simulink model "Part1_170747"  (R2019a)
settings: Solver=ode2  StartTime=0.0  StopTime=700  FixedStep=0.1  RelTol=1e-3
undefined symbols (not defined in the file): D, Km, T
settings Model: Creator=HP  LastModifiedBy=singh
settings DataIOCC: ReturnWorkspaceOutputs=off
settings DebuggingCC: ArithmeticOperatorsInVariantConditions=warning

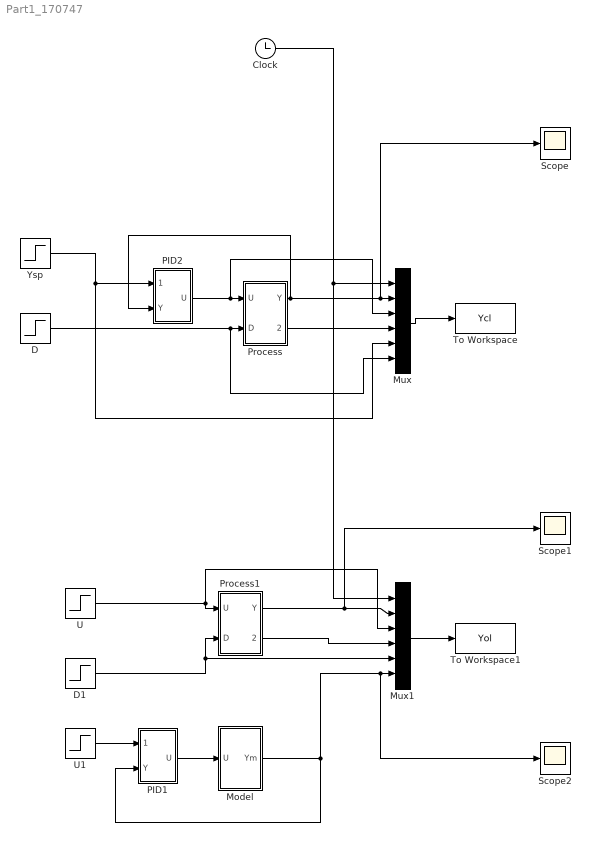
== system Part1_170747 ==
  Clock : Clock
  D : Step  Time=0  After=0  SampleTime=0
  D1 : Step  Time=0  After=0  SampleTime=0
  Model : Subsystem
  Mux : Mux  Inputs=6
  Mux1 : Mux  Inputs=6
  PID1 : Subsystem  mask{Kc=2.81, Ti=1e10, Td=0}
      mask prompts: Kc "Proportional Gain"; Ti "Integral Time"; Td "Derivative Time"
  PID2 : Subsystem  mask{Kc=3.4071/1.7, Ti=106.2/2, Td=106.2/8}
      mask prompts: Kc "Proportional Gain"; Ti "Integral Time"; Td "Derivative Time"
  Process : Subsystem  mask{K1=0.45, K2=0.45, T1=0.5, T2=0.5, K=1/17e-4}
      mask prompts: K1 "Forward Gain"; K2 "Rev Gain"; T1 "Forward Time Constt"; T2 "Rev Time Constt"; K "Scaling Gain"
  Process1 : Subsystem  mask{K1=0.45, K2=0.45, T1=0.5, T2=0.5, K=1/17e-4}
      mask prompts: K1 "Forward Gain"; K2 "Rev Gain"; T1 "Forward Time Constt"; T2 "Rev Time Constt"; K "Scaling Gain"
  Scope : Scope
  Scope1 : Scope
  Scope2 : Scope
  To Workspace : ToWorkspace  VariableName=Ycl  SampleTime=-1
  To Workspace1 : ToWorkspace  VariableName=Yol  SampleTime=-1
  U : Step  Time=0  SampleTime=0
  U1 : Step  Time=0  SampleTime=0
  Ysp : Step  Time=0  SampleTime=0
  wires:
  Clock/1 -> Mux/1, Mux1/1
  Process/1(Y) -> PID2/2(Y), Scope/1, Mux/2
  Process/2(Uimp) -> Mux/4
  Mux/1 -> To Workspace/1
  D/1 -> Mux/6, Process/2(D)
  Ysp/1 -> PID2/1(Ysp), Mux/5
  Mux1/1 -> To Workspace1/1
  U/1 -> Mux1/3, Process1/1(U)
  D1/1 -> Process1/2(D), Mux1/5
  Process1/1(Y) -> Mux1/2, Scope1/1
  PID2/1(U) -> Mux/3, Process/1(U)
  Process1/2(Uimp) -> Mux1/4
  Model/1("Ym ") -> Scope2/1, Mux1/6, PID1/2(Y)
  PID1/1(U) -> Model/1(U)
  U1/1 -> PID1/1(Ysp)

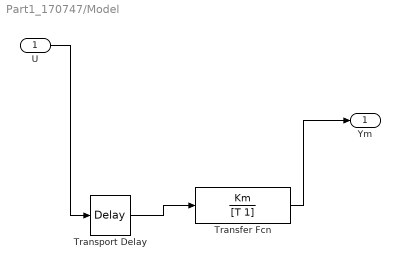
== system Part1_170747/Model ==
  U : Inport
  Transfer Fcn : TransferFcn  Numerator=Km  Denominator=[T 1]
  Transport Delay : TransportDelay  DelayTime=D
  "Ym " : Outport
  wires:
  Transport Delay/1 -> Transfer Fcn/1
  Transfer Fcn/1 -> "Ym "/1
  U/1 -> Transport Delay/1

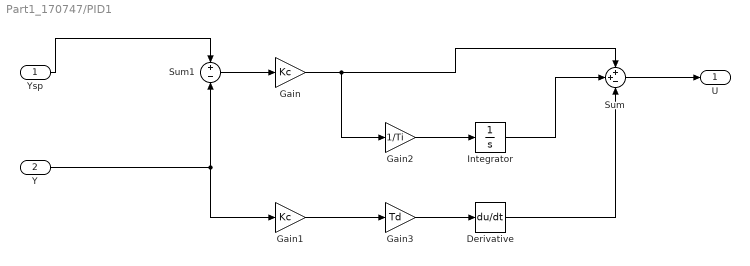
== system Part1_170747/PID1 ==
  Ysp : Inport
  Y : Inport  Port=2
  Derivative : Derivative
  Gain : Gain  Gain=Kc
  Gain1 : Gain  Gain=Kc
  Gain2 : Gain  Gain=1/Ti
  Gain3 : Gain  Gain=Td
  Integrator : Integrator
  Sum : Sum  Inputs=++-
  Sum1 : Sum  Inputs=+-
  U : Outport
  wires:
  Sum1/1 -> Gain/1
  Y/1 -> Gain1/1, Sum1/2
  Gain2/1 -> Integrator/1
  Gain/1 -> Gain2/1, Sum/1
  Integrator/1 -> Sum/2
  Derivative/1 -> Sum/3
  Gain3/1 -> Derivative/1
  Sum/1 -> U/1
  Gain1/1 -> Gain3/1
  Ysp/1 -> Sum1/1

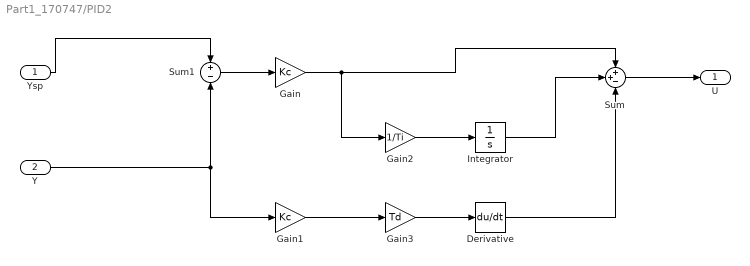
== system Part1_170747/PID2 ==
  Ysp : Inport
  Y : Inport  Port=2
  Derivative : Derivative
  Gain : Gain  Gain=Kc
  Gain1 : Gain  Gain=Kc
  Gain2 : Gain  Gain=1/Ti
  Gain3 : Gain  Gain=Td
  Integrator : Integrator
  Sum : Sum  Inputs=++-
  Sum1 : Sum  Inputs=+-
  U : Outport
  wires:
  Sum1/1 -> Gain/1
  Y/1 -> Gain1/1, Sum1/2
  Gain2/1 -> Integrator/1
  Gain/1 -> Gain2/1, Sum/1
  Integrator/1 -> Sum/2
  Derivative/1 -> Sum/3
  Gain3/1 -> Derivative/1
  Sum/1 -> U/1
  Gain1/1 -> Gain3/1
  Ysp/1 -> Sum1/1

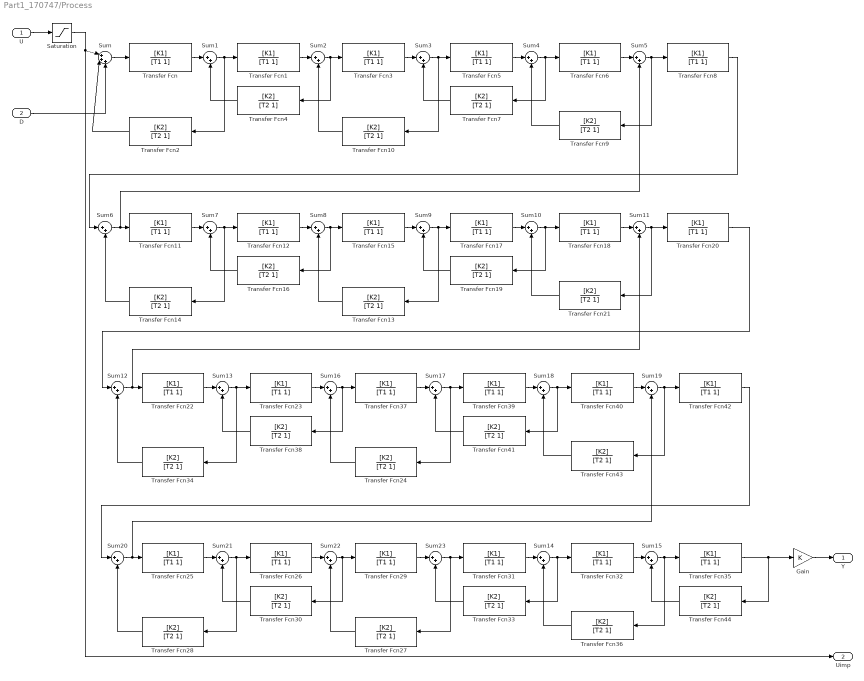
== system Part1_170747/Process ==
  U : Inport
  D : Inport  Port=2
  Gain : Gain  Gain=K
  Saturation : Saturate  UpperLimit=10  LowerLimit=-10
  Sum : Sum  Inputs=|+++
  Sum{1..23} (23 alike) : Sum  Inputs=|++
  Transfer Fcn{,1,3,5..6,8,11..12,15,17..18,20,22..23,25..26,29,31..32,35,37,39..40,42} (24 alike) : TransferFcn  Numerator=[K1]  Denominator=[T1 1]
  Transfer Fcn{2,4,7,9..10,13..14,16,19,21,24,27..28,30,33..34,36,38,41,43..44} (21 alike) : TransferFcn  Numerator=[K2]  Denominator=[T2 1]
  Y : Outport
  Uimp : Outport  Port=2
  wires:
  Transfer Fcn14/1 -> Sum6/2
  Transfer Fcn13/1 -> Sum8/2
  Transfer Fcn18/1 -> Sum11/1
  Transfer Fcn1/1 -> Sum2/1
  Sum18/1 -> Transfer Fcn41/1, Transfer Fcn40/1
  Sum21/1 -> Transfer Fcn28/1, Transfer Fcn26/1
  Transfer Fcn26/1 -> Sum22/1
  Transfer Fcn15/1 -> Sum9/1
  Sum13/1 -> Transfer Fcn34/1, Transfer Fcn23/1
  Sum7/1 -> Transfer Fcn14/1, Transfer Fcn12/1
  Sum8/1 -> Transfer Fcn16/1, Transfer Fcn15/1
  Transfer Fcn20/1 -> Sum12/1
  Sum20/1 -> Sum19/2, Transfer Fcn25/1
  Transfer Fcn9/1 -> Sum4/2
  Transfer Fcn25/1 -> Sum21/1
  Sum12/1 -> Sum11/2, Transfer Fcn22/1
  Transfer Fcn12/1 -> Sum8/1
  Transfer Fcn16/1 -> Sum7/2
  Transfer Fcn44/1 -> Sum15/2
  Transfer Fcn39/1 -> Sum18/1
  Sum2/1 -> Transfer Fcn4/1, Transfer Fcn3/1
  Transfer Fcn38/1 -> Sum13/2
  Sum17/1 -> Transfer Fcn24/1, Transfer Fcn39/1
  Sum9/1 -> Transfer Fcn13/1, Transfer Fcn17/1
  D/1 -> Sum/3
  Transfer Fcn35/1 -> Gain/1, Transfer Fcn44/1
  Sum11/1 -> Transfer Fcn21/1, Transfer Fcn20/1
  Transfer Fcn42/1 -> Sum20/1
  Sum1/1 -> Transfer Fcn2/1, Transfer Fcn1/1
  Sum15/1 -> Transfer Fcn36/1, Transfer Fcn35/1
  Transfer Fcn27/1 -> Sum22/2
  Transfer Fcn24/1 -> Sum16/2
  Transfer Fcn31/1 -> Sum14/1
  Transfer Fcn23/1 -> Sum16/1
  Sum14/1 -> Transfer Fcn33/1, Transfer Fcn32/1
  Sum23/1 -> Transfer Fcn27/1, Transfer Fcn31/1
  Transfer Fcn40/1 -> Sum19/1
  Sum16/1 -> Transfer Fcn38/1, Transfer Fcn37/1
  Transfer Fcn22/1 -> Sum13/1
  Transfer Fcn34/1 -> Sum12/2
  Transfer Fcn37/1 -> Sum17/1
  Transfer Fcn33/1 -> Sum23/2
  Transfer Fcn41/1 -> Sum17/2
  Sum4/1 -> Transfer Fcn7/1, Transfer Fcn6/1
  Transfer Fcn36/1 -> Sum14/2
  Sum10/1 -> Transfer Fcn19/1, Transfer Fcn18/1
  Sum22/1 -> Transfer Fcn30/1, Transfer Fcn29/1
  Transfer Fcn6/1 -> Sum5/1
  Transfer Fcn29/1 -> Sum23/1
  Transfer Fcn2/1 -> Sum/2
  Transfer Fcn28/1 -> Sum20/2
  Transfer Fcn17/1 -> Sum10/1
  Transfer Fcn30/1 -> Sum21/2
  Transfer Fcn43/1 -> Sum18/2
  Transfer Fcn5/1 -> Sum4/1
  Sum19/1 -> Transfer Fcn43/1, Transfer Fcn42/1
  Sum3/1 -> Transfer Fcn10/1, Transfer Fcn5/1
  Transfer Fcn32/1 -> Sum15/1
  Sum6/1 -> Sum5/2, Transfer Fcn11/1
  Transfer Fcn/1 -> Sum1/1
  Transfer Fcn21/1 -> Sum10/2
  Sum5/1 -> Transfer Fcn9/1, Transfer Fcn8/1
  Transfer Fcn7/1 -> Sum3/2
  Transfer Fcn4/1 -> Sum1/2
  Transfer Fcn11/1 -> Sum7/1
  Transfer Fcn10/1 -> Sum2/2
  Transfer Fcn3/1 -> Sum3/1
  Transfer Fcn8/1 -> Sum6/1
  Transfer Fcn19/1 -> Sum9/2
  Sum/1 -> Transfer Fcn/1
  Gain/1 -> Y/1
  U/1 -> Saturation/1
  Saturation/1 -> Uimp/1, Sum/1

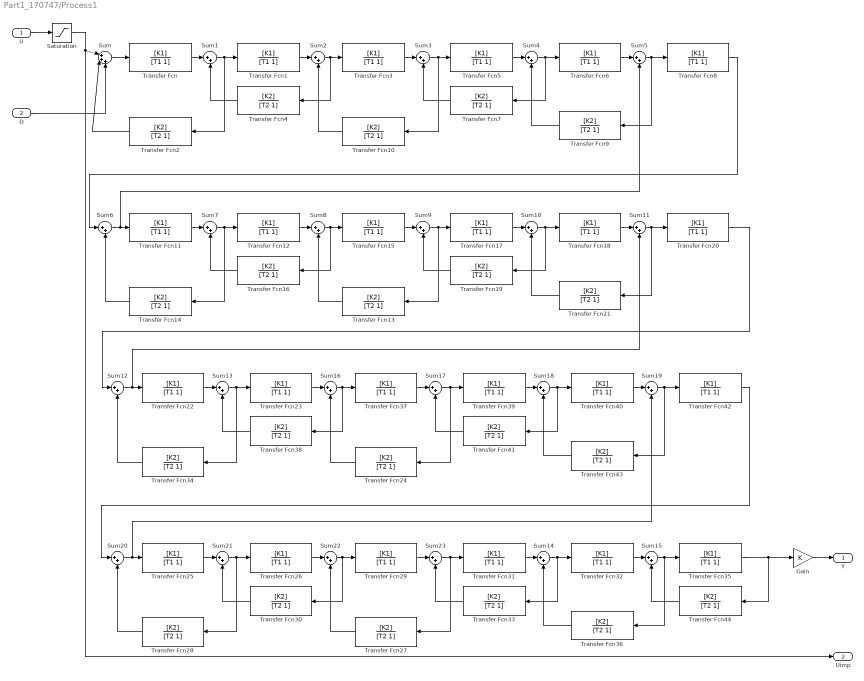
== system Part1_170747/Process1 ==
  U : Inport
  D : Inport  Port=2
  Gain : Gain  Gain=K
  Saturation : Saturate  UpperLimit=10  LowerLimit=-10
  Sum : Sum  Inputs=|+++
  Sum{1..23} (23 alike) : Sum  Inputs=|++
  Transfer Fcn{,1,3,5..6,8,11..12,15,17..18,20,22..23,25..26,29,31..32,35,37,39..40,42} (24 alike) : TransferFcn  Numerator=[K1]  Denominator=[T1 1]
  Transfer Fcn{2,4,7,9..10,13..14,16,19,21,24,27..28,30,33..34,36,38,41,43..44} (21 alike) : TransferFcn  Numerator=[K2]  Denominator=[T2 1]
  Y : Outport
  Uimp : Outport  Port=2
  wires:
  Transfer Fcn14/1 -> Sum6/2
  Transfer Fcn13/1 -> Sum8/2
  Transfer Fcn18/1 -> Sum11/1
  Transfer Fcn1/1 -> Sum2/1
  Sum18/1 -> Transfer Fcn41/1, Transfer Fcn40/1
  Sum21/1 -> Transfer Fcn28/1, Transfer Fcn26/1
  Transfer Fcn26/1 -> Sum22/1
  Transfer Fcn15/1 -> Sum9/1
  Sum13/1 -> Transfer Fcn34/1, Transfer Fcn23/1
  Sum7/1 -> Transfer Fcn14/1, Transfer Fcn12/1
  Sum8/1 -> Transfer Fcn16/1, Transfer Fcn15/1
  Transfer Fcn20/1 -> Sum12/1
  Sum20/1 -> Sum19/2, Transfer Fcn25/1
  Transfer Fcn9/1 -> Sum4/2
  Transfer Fcn25/1 -> Sum21/1
  Sum12/1 -> Sum11/2, Transfer Fcn22/1
  Transfer Fcn12/1 -> Sum8/1
  Transfer Fcn16/1 -> Sum7/2
  Transfer Fcn44/1 -> Sum15/2
  Transfer Fcn39/1 -> Sum18/1
  Sum2/1 -> Transfer Fcn4/1, Transfer Fcn3/1
  Transfer Fcn38/1 -> Sum13/2
  Sum17/1 -> Transfer Fcn24/1, Transfer Fcn39/1
  Sum9/1 -> Transfer Fcn13/1, Transfer Fcn17/1
  D/1 -> Sum/3
  Transfer Fcn35/1 -> Gain/1, Transfer Fcn44/1
  Sum11/1 -> Transfer Fcn21/1, Transfer Fcn20/1
  Transfer Fcn42/1 -> Sum20/1
  Sum1/1 -> Transfer Fcn2/1, Transfer Fcn1/1
  Sum15/1 -> Transfer Fcn36/1, Transfer Fcn35/1
  Transfer Fcn27/1 -> Sum22/2
  Transfer Fcn24/1 -> Sum16/2
  Transfer Fcn31/1 -> Sum14/1
  Transfer Fcn23/1 -> Sum16/1
  Sum14/1 -> Transfer Fcn33/1, Transfer Fcn32/1
  Sum23/1 -> Transfer Fcn27/1, Transfer Fcn31/1
  Transfer Fcn40/1 -> Sum19/1
  Sum16/1 -> Transfer Fcn38/1, Transfer Fcn37/1
  Transfer Fcn22/1 -> Sum13/1
  Transfer Fcn34/1 -> Sum12/2
  Transfer Fcn37/1 -> Sum17/1
  Transfer Fcn33/1 -> Sum23/2
  Transfer Fcn41/1 -> Sum17/2
  Sum4/1 -> Transfer Fcn7/1, Transfer Fcn6/1
  Transfer Fcn36/1 -> Sum14/2
  Sum10/1 -> Transfer Fcn19/1, Transfer Fcn18/1
  Sum22/1 -> Transfer Fcn30/1, Transfer Fcn29/1
  Transfer Fcn6/1 -> Sum5/1
  Transfer Fcn29/1 -> Sum23/1
  Transfer Fcn2/1 -> Sum/2
  Transfer Fcn28/1 -> Sum20/2
  Transfer Fcn17/1 -> Sum10/1
  Transfer Fcn30/1 -> Sum21/2
  Transfer Fcn43/1 -> Sum18/2
  Transfer Fcn5/1 -> Sum4/1
  Sum19/1 -> Transfer Fcn43/1, Transfer Fcn42/1
  Sum3/1 -> Transfer Fcn10/1, Transfer Fcn5/1
  Transfer Fcn32/1 -> Sum15/1
  Sum6/1 -> Sum5/2, Transfer Fcn11/1
  Transfer Fcn/1 -> Sum1/1
  Transfer Fcn21/1 -> Sum10/2
  Sum5/1 -> Transfer Fcn9/1, Transfer Fcn8/1
  Transfer Fcn7/1 -> Sum3/2
  Transfer Fcn4/1 -> Sum1/2
  Transfer Fcn11/1 -> Sum7/1
  Transfer Fcn10/1 -> Sum2/2
  Transfer Fcn3/1 -> Sum3/1
  Transfer Fcn8/1 -> Sum6/1
  Transfer Fcn19/1 -> Sum9/2
  Sum/1 -> Transfer Fcn/1
  Gain/1 -> Y/1
  U/1 -> Saturation/1
  Saturation/1 -> Uimp/1, Sum/1
